simulink model "verification"  (R2015b)
settings: Solver=VariableStepAuto  StartTime=0.0  StopTime=inf  RelTol=1e-3
libraries: neural x20, visionsinks x2, visionstatistics x1
(part 1 of 3)
settings Model: Creator=User  LastModifiedBy=User

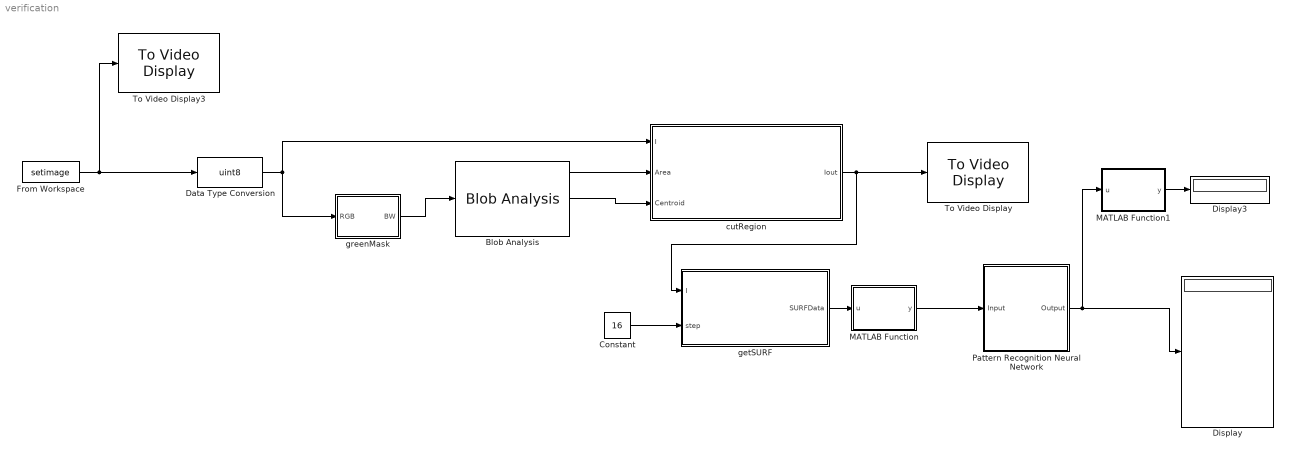
== system verification ==
  Blob Analysis : visionstatistics/Blob Analysis  Tag=vipblks_row_conv  area=on  centroid=on  bBox=on  majorAxis=off  minorAxis=off  angle=off  eccentricity=off  equivDiameterSq=off  extent=off  perimeter=off  maxBlobs=10  warnIfNumBlobsExceeded=on  isCount=off  useMinArea=off  minArea=0  useMaxArea=off  maxArea=intmax('uint32')  excludeBorderBlob=off  outDT=double  isOutVarDim=off  isFill=on  fillValues=-1  conn=8  isLabel=off  outputMode=Binary point scaling  outputWordLength=32  outputFracLength=16  firstCoeffMode=Binary point scaling  firstCoeffWordLength=16  firstCoeffFracLength=14  secondCoeffMode=Binary point scaling  secondCoeffWordLength=32  secondCoeffFracLength=16  accumMode=Binary point scaling  accumWordLength=32  accumFracLength=0  prodOutputMode=Binary point scaling  prodOutputWordLength=32  prodOutputFracLength=16  roundingMode=Floor  overflowMode=off
  Constant : Constant  Value=16
  Data Type Conversion : DataTypeConversion  OutDataTypeStr=uint8
  Display : Display
  Display3 : Display
  From Workspace : FromWorkspace  VariableName=setimage  SampleTime=2  Interpolate=off  OutputAfterFinalValue=Setting to zero
  MATLAB Function : MATLAB Function  TreatAsAtomicUnit=on
  MATLAB Function1 : MATLAB Function  TreatAsAtomicUnit=on
  Pattern Recognition Neural Network : Subsystem
      mask help: Pattern Recognition Neural Network
      mask Display: e = 0.06;c1 = [120 150 230]/255;c2 = ([120 150 230]+0)/383;c3 = ([120 150 230]+128)/383;patch([0 1 1 0],[0 0 1 1],c1);patch([0 1 1 1-e 1-e 0+e],[0 0 1 1-e 0+e 0+e],c2);patch([0 0 1 1-e 0+e 0+e],[0 1 1 1-e 1-e 0+e],c3);plot([0 1 1 0 0],[0 0 1 1 0]);fprintf('NNET');port_label('input',1,' Input');port_label('output',1,'Output ');
  To Video Display : visionsinks/To Video Display  windowSizeMode=Normal  openAtMdlStart=on  fullScreen=off  videoWindowX=1478  videoWindowY=273  saveWindowSize=off  videoWindowWidth=160  videoWindowHeight=160  inputColorFormat=RGB  inputType=Obsolete  imagePorts=One multidimensional signal  OutputDevice=On-screen video monitor  dataOrg=Column-major  isWindowOpen=off
  To Video Display3 : visionsinks/To Video Display  windowSizeMode=Normal  openAtMdlStart=on  fullScreen=off  videoWindowX=536805376  videoWindowY=536805376  saveWindowSize=off  videoWindowWidth=2147483647  videoWindowHeight=2147483647  inputColorFormat=RGB  inputType=Obsolete  imagePorts=One multidimensional signal  OutputDevice=On-screen video monitor  dataOrg=Column-major  isWindowOpen=off
  cutRegion : MATLAB Function  TreatAsAtomicUnit=on
  getSURF : MATLAB Function  TreatAsAtomicUnit=on
  greenMask : MATLAB Function  TreatAsAtomicUnit=on
  wires:
  greenMask/1(BW) -> Blob Analysis/1
  Blob Analysis/2 -> cutRegion/3(Centroid)
  Blob Analysis/1 -> cutRegion/2(Area)
  Constant/1 -> getSURF/2(step)
  cutRegion/1(Iout) -> To Video Display/1, getSURF/1(I)
  Data Type Conversion/1 -> cutRegion/1(I), greenMask/1(RGB)
  getSURF/1(SURFData) -> MATLAB Function/1(u)
  MATLAB Function/1(y) -> Pattern Recognition Neural Network/1(Input)
  From Workspace/1 -> To Video Display3/1, Data Type Conversion/1
  Pattern Recognition Neural Network/1(Output) -> MATLAB Function1/1(u), Display/1
  MATLAB Function1/1(y) -> Display3/1

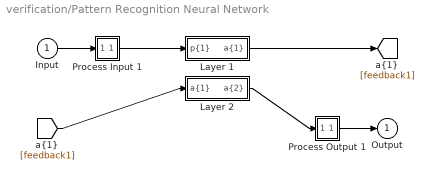
== system verification/Pattern Recognition Neural Network ==
  Input : Inport  PortDimensions=349
      mask Display: e = 0.06;c1 = [120 230 180]/255;c2 = ([120 230 180]+0)/(256+128);c3 = ([120 230 180]+128)/(256+128);patch([0 1 1 0],[0 0 1 1],c1);patch([0 1 1 1-e 1-e 0+e],[0 0 1 1-e 0+e 0+e],c2);patch([0 0 1 1-e 0+e 0+e],[0 1 1 1-e 1-e 0+e],c3);plot([0 1 1 0 0],[0 0 1 1 0]);
  Layer 1 : Subsystem
      mask Display: e = 0.06;c1 = [120 150 230]/255;c2 = ([120 150 230]+0)/383;c3 = ([120 150 230]+128)/383;patch([0 1 1 0],[0 0 1 1],c1);patch([0 1 1 1-e 1-e 0+e],[0 0 1 1-e 0+e 0+e],c2);patch([0 0 1 1-e 0+e 0+e],[0 1 1 1-e 1-e 0+e],c3);plot([0 1 1 0 0],[0 0 1 1 0]);
  Layer 2 : Subsystem
      mask Display: e = 0.06;c1 = [120 150 230]/255;c2 = ([120 150 230]+0)/383;c3 = ([120 150 230]+128)/383;patch([0 1 1 0],[0 0 1 1],c1);patch([0 1 1 1-e 1-e 0+e],[0 0 1 1-e 0+e 0+e],c2);patch([0 0 1 1-e 0+e 0+e],[0 1 1 1-e 1-e 0+e],c3);plot([0 1 1 0 0],[0 0 1 1 0]);
  Process Input 1 : Subsystem
      mask Display: e = 0.06;c1 = [120 150 230]/255;c2 = ([120 150 230]+0)/383;c3 = ([120 150 230]+128)/383;patch([0 1 1 0],[0 0 1 1],c1);patch([0 1 1 1-e 1-e 0+e],[0 0 1 1-e 0+e 0+e],c2);patch([0 0 1 1-e 0+e 0+e],[0 1 1 1-e 1-e 0+e],c3);plot([0 1 1 0 0],[0 0 1 1 0]);
  Process Output 1 : Subsystem
      mask Display: e = 0.06;c1 = [120 150 230]/255;c2 = ([120 150 230]+0)/383;c3 = ([120 150 230]+128)/383;patch([0 1 1 0],[0 0 1 1],c1);patch([0 1 1 1-e 1-e 0+e],[0 0 1 1-e 0+e 0+e],c2);patch([0 0 1 1-e 0+e 0+e],[0 1 1 1-e 1-e 0+e],c3);plot([0 1 1 0 0],[0 0 1 1 0]);
  Output : Outport  InitialOutput=[0;0;0;0;0;0;0]
      mask Display: e = 0.06;c1 = [120 230 180]/255;c2 = ([120 230 180]+0)/(256+128);c3 = ([120 230 180]+128)/(256+128);patch([0 1 1 0],[0 0 1 1],c1);patch([0 1 1 1-e 1-e 0+e],[0 0 1 1-e 0+e 0+e],c2);patch([0 0 1 1-e 0+e 0+e],[0 1 1 1-e 1-e 0+e],c3);plot([0 1 1 0 0],[0 0 1 1 0]);
  wires:
  Input/1 -> Process Input 1/1(x)
  Process Output 1/1(y) -> Output/1
  Process Input 1/1(p) -> Layer 1/1("p{1}")
  Layer 1/1("a{1}") -> [feedback1]
  [feedback1] -> Layer 2/1("a{1} ")
  Layer 2/1("a{2}") -> Process Output 1/1(a)

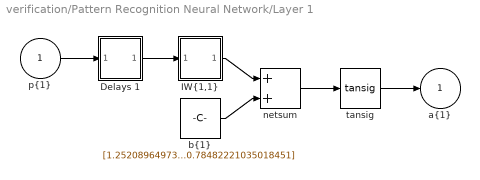
== system verification/Pattern Recognition Neural Network/Layer 1 ==
  "p{1}" : Inport  PortDimensions=349
      mask Display: e = 0.06;c1 = [120 230 180]/255;c2 = ([120 230 180]+0)/(256+128);c3 = ([120 230 180]+128)/(256+128);patch([0 1 1 0],[0 0 1 1],c1);patch([0 1 1 1-e 1-e 0+e],[0 0 1 1-e 0+e 0+e],c2);patch([0 0 1 1-e 0+e 0+e],[0 1 1 1-e 1-e 0+e],c3);plot([0 1 1 0 0],[0 0 1 1 0]);
  Delays 1 : Subsystem
      mask Display: e = 0.06;c1 = [120 150 230]/255;c2 = ([120 150 230]+0)/383;c3 = ([120 150 230]+128)/383;patch([0 1 1 0],[0 0 1 1],c1);patch([0 1 1 1-e 1-e 0+e],[0 0 1 1-e 0+e 0+e],c2);patch([0 0 1 1-e 0+e 0+e],[0 1 1 1-e 1-e 0+e],c3);plot([0 1 1 0 0],[0 0 1 1 0]);disp('0');
  "IW{1,1}" : Subsystem
      mask Display: e = 0.06;c1 = [120 150 230]/255;c2 = ([120 150 230]+0)/383;c3 = ([120 150 230]+128)/383;patch([0 1 1 0],[0 0 1 1],c1);patch([0 1 1 1-e 1-e 0+e],[0 0 1 1-e 0+e 0+e],c2);patch([0 0 1 1-e 0+e 0+e],[0 1 1 1-e 1-e 0+e],c3);plot([0 1 1 0 0],[0 0 1 1 0]);disp('W');
  "b{1}" : Constant  Value=[1.2520896497359288;-0.92281616914926501;-1.5755720804159823;-0.48231286693993536;0.032429505453323522;-0.10257136982966432;0.079130367651085678;0.67536543039361374;0.53417313742188333;0.78482221035018451]
      mask Display: e = 0.06;c1 = [120 150 230]/255;c2 = ([120 150 230]+0)/383;c3 = ([120 150 230]+128)/383;patch([0 1 1 0],[0 0 1 1],c1);patch([0 1 1 1-e 1-e 0+e],[0 0 1 1-e 0+e 0+e],c2);patch([0 0 1 1-e 0+e 0+e],[0 1 1 1-e 1-e 0+e],c3);plot([0 1 1 0 0],[0 0 1 1 0]);disp('b');
  netsum : Sum  Inputs=2  SaturateOnIntegerOverflow=on  InputSameDT=on  OutDataTypeStr=Inherit: Same as first input
      mask Display: e = 0.06;c1 = [120 150 230]/255;c2 = ([120 150 230]+0)/383;c3 = ([120 150 230]+128)/383;patch([0 1 1 0],[0 0 1 1],c1);patch([0 1 1 1-e 1-e 0+e],[0 0 1 1-e 0+e 0+e],c2);patch([0 0 1 1-e 0+e 0+e],[0 1 1 1-e 1-e 0+e],c3);plot([0 1 1 0 0],[0 0 1 1 0]);disp('+');
  tansig : neural/Transfer Functions/tansig
  "a{1}" : Outport  InitialOutput=[0;0;0;0;0;0;0;0;0;0]
      mask Display: e = 0.06;c1 = [120 230 180]/255;c2 = ([120 230 180]+0)/(256+128);c3 = ([120 230 180]+128)/(256+128);patch([0 1 1 0],[0 0 1 1],c1);patch([0 1 1 1-e 1-e 0+e],[0 0 1 1-e 0+e 0+e],c2);patch([0 0 1 1-e 0+e 0+e],[0 1 1 1-e 1-e 0+e],c3);plot([0 1 1 0 0],[0 0 1 1 0]);
  wires:
  "p{1}"/1 -> Delays 1/1("p{1}")
  Delays 1/1("pd{1,1}") -> "IW{1,1}"/1("pd{1,1}")
  "IW{1,1}"/1("iz{1,1}") -> netsum/1
  "b{1}"/1 -> netsum/2
  netsum/1 -> tansig/1
  tansig/1 -> "a{1}"/1

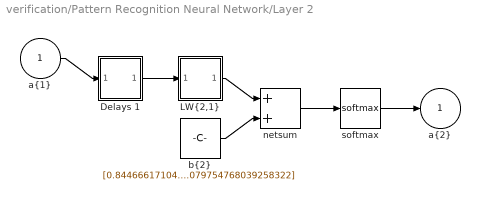
== system verification/Pattern Recognition Neural Network/Layer 2 ==
  "a{1} " : Inport  PortDimensions=10
      mask Display: e = 0.06;c1 = [120 230 180]/255;c2 = ([120 230 180]+0)/(256+128);c3 = ([120 230 180]+128)/(256+128);patch([0 1 1 0],[0 0 1 1],c1);patch([0 1 1 1-e 1-e 0+e],[0 0 1 1-e 0+e 0+e],c2);patch([0 0 1 1-e 0+e 0+e],[0 1 1 1-e 1-e 0+e],c3);plot([0 1 1 0 0],[0 0 1 1 0]);
  Delays 1 : Subsystem
      mask Display: e = 0.06;c1 = [120 150 230]/255;c2 = ([120 150 230]+0)/383;c3 = ([120 150 230]+128)/383;patch([0 1 1 0],[0 0 1 1],c1);patch([0 1 1 1-e 1-e 0+e],[0 0 1 1-e 0+e 0+e],c2);patch([0 0 1 1-e 0+e 0+e],[0 1 1 1-e 1-e 0+e],c3);plot([0 1 1 0 0],[0 0 1 1 0]);disp('0');
  "LW{2,1}" : Subsystem
      mask Display: e = 0.06;c1 = [120 150 230]/255;c2 = ([120 150 230]+0)/383;c3 = ([120 150 230]+128)/383;patch([0 1 1 0],[0 0 1 1],c1);patch([0 1 1 1-e 1-e 0+e],[0 0 1 1-e 0+e 0+e],c2);patch([0 0 1 1-e 0+e 0+e],[0 1 1 1-e 1-e 0+e],c3);plot([0 1 1 0 0],[0 0 1 1 0]);disp('W');
  "b{2}" : Constant  Value=[0.8446661710451735;-0.96183712929880982;0.74210025390233625;0.16753901818095251;-0.54254157655283242;-0.63817454211815539;-0.079754768039258322]
      mask Display: e = 0.06;c1 = [120 150 230]/255;c2 = ([120 150 230]+0)/383;c3 = ([120 150 230]+128)/383;patch([0 1 1 0],[0 0 1 1],c1);patch([0 1 1 1-e 1-e 0+e],[0 0 1 1-e 0+e 0+e],c2);patch([0 0 1 1-e 0+e 0+e],[0 1 1 1-e 1-e 0+e],c3);plot([0 1 1 0 0],[0 0 1 1 0]);disp('b');
  netsum : Sum  Inputs=2  SaturateOnIntegerOverflow=on  InputSameDT=on  OutDataTypeStr=Inherit: Same as first input
      mask Display: e = 0.06;c1 = [120 150 230]/255;c2 = ([120 150 230]+0)/383;c3 = ([120 150 230]+128)/383;patch([0 1 1 0],[0 0 1 1],c1);patch([0 1 1 1-e 1-e 0+e],[0 0 1 1-e 0+e 0+e],c2);patch([0 0 1 1-e 0+e 0+e],[0 1 1 1-e 1-e 0+e],c3);plot([0 1 1 0 0],[0 0 1 1 0]);disp('+');
  softmax : neural/Transfer Functions/softmax
  "a{2}" : Outport  InitialOutput=[0;0;0;0;0;0;0]
      mask Display: e = 0.06;c1 = [120 230 180]/255;c2 = ([120 230 180]+0)/(256+128);c3 = ([120 230 180]+128)/(256+128);patch([0 1 1 0],[0 0 1 1],c1);patch([0 1 1 1-e 1-e 0+e],[0 0 1 1-e 0+e 0+e],c2);patch([0 0 1 1-e 0+e 0+e],[0 1 1 1-e 1-e 0+e],c3);plot([0 1 1 0 0],[0 0 1 1 0]);
  wires:
  "a{1} "/1 -> Delays 1/1("p{2}")
  Delays 1/1("pd{2,1}") -> "LW{2,1}"/1("ad{2,1}")
  "LW{2,1}"/1("lz{2,1}") -> netsum/1
  "b{2}"/1 -> netsum/2
  netsum/1 -> softmax/1
  softmax/1 -> "a{2}"/1

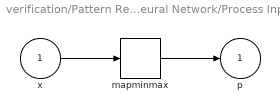
== system verification/Pattern Recognition Neural Network/Process Input 1 ==
  x : Inport  PortDimensions=349
      mask Display: e = 0.06;c1 = [120 230 180]/255;c2 = ([120 230 180]+0)/(256+128);c3 = ([120 230 180]+128)/(256+128);patch([0 1 1 0],[0 0 1 1],c1);patch([0 1 1 1-e 1-e 0+e],[0 0 1 1-e 0+e 0+e],c2);patch([0 0 1 1-e 0+e 0+e],[0 1 1 1-e 1-e 0+e],c3);plot([0 1 1 0 0],[0 0 1 1 0]);
  mapminmax : neural/Processing Functions/mapminmax  xmin=[-11129.965961101443;1134.6567206044926;-2376.3659908917143;-4334.0372445314288;7757.4027746883612;-6984.4334074929839;-2777.9527058342687;3155.9690581192376;-1330.691241389575;4257.0589253908138;-623.20684359631468;-2001.566675005465;-4932.7134689911391;304.46851647603125;-967.32875854233816;640.73136885648694;386.66074504769114;1002.1623313175693;-3184.007659381773;-381.37803132283284;-3295.858092291508;-1489.0871261009588;-226.49555101296443;-2405.8867516242576;-2776.7794520500211;-1541.0170324268913;101.43967602768807;-100.76443127754578;-593.03637636096903;1357.9634170740264;1407.3950263055601;-483.66947575357494;-1889.9176508706948;-1629.3955251451089;-726.50327548468738;-1853.6072505650598;-1498.8553267377129;-1530.3633390778268;268.18750457084093;-2240.9999713540606;-1598.6795958119494;-1582.907954987654;380.23677697560817;-687.57622036680209;-2158.6653002343019;-1530.8506902527345;-2225.7407166340577;-1737.1719827748605;386.28554587051292;-2047.1309669819805;-1417.8656347977224;-612.48056407820786;676.45691636688923;446.38920725912357;74.470862862096908;39.174713487048386;-1007.1653257389228;-1067.5381147129376;-1589.7717010748245;369.32541111978048;-15.568258331743834;-2618.166478036178;66.851725230876625;-2632.6489110914567;-152.27189245653938;-961.70356716324886;-68.16047275108798;-1389.6973712632755;-1544.6280829615475;-1078.1701102250183;-1083.2475056257147;-70.327106602471815;-1389.6912572643412;-501.87203323128261;-1211.1299730501946;-873.8563577745025;135.23078707803614;510.40761207152661;67.976583540881691;-382.71067889430486;-2440.8434161611667;-960.30021713058647;601.55410753465776;-920.69305223222057;-945.98625046016025;-1158.0540952187496;260.30244378313034;-1087.9748915817286;-582.19629937786613;-494.80610196790803;-1423.8822861380806;-1415.6427970118482;-589.82126941908848;66.389992254750979;-1287.5678718628087;-40.246203034889106;-1450.5155667211093;-697.93893844304534;-121.38825064237872;-1029.850343236707;-258.78167810452703;-1184.1571756240155;-175.02600935248478;-1173.3831276484862;-845.55385054668193;-1118.0261569261522;-112.80399351655041;285.29099479332041;-406.88257108720899;-824.4577050291407;-913.16225540445407;-431.74577653476297;-535.29039798765666;-559.55309131633362;-859.66088958315208;-1382.5184253003295;-634.44889621500624;-869.9885065509344;-1736.0447306117053;-989.43057866603237;-377.04364635953357;-655.34244197384805;-1161.4001166516846;-354.69697407530305;-410.240777822631;-763.08944947808925;-882.01049096338215;-17.297235561955929;-853.68060261106541;-388.55640302193973;260.40063239144388;-614.33797117366726;-1166.0372444888003;-829.31885826600205;-1106.1198195175425;-117.14159077934548;172.43508067231105;-269.31758186795628;-1189.4586228827602;-585.82582165939368;-296.54465016092115;-1217.9356712043461;-425.125346288532;-956.89102108175575;130.81562066503227;-650.61070961528071;-35.453495601084455;-374.16957679196389;-756.19410654695184;-436.24479084948632;-166.7746883075414;-402.54135427924291;-1012.3923778324571;-448.67046874191061;-288.18820186606865;-99.014151169624313;-160.80695606286076;-521.75050070627856;-565.41663842242019;-576.59406290264189;-778.2488779178459;-1366.4710747970648;-368.11986679262969;-470.81863934027433;-314.58819838502666;-766.97148873280241;-468.21981709565682;-120.09837788639067;-936.80795693703726;-574.10147881344369;-556.44364225382867;-101.95169318831634;-292.5992032047817;-1077.7752146961855;461.34208371091569;492.30461418312234;-62.101593456599197;-277.72177129517496;-715.16524137409272;-820.91429927317392;-403.25066908313806;-354.19848681396775;-328.28100657612879;-606.65121012463112;-723.6632390586019;-126.01168221322104;496.64864785796067;-527.94553740683682;-76.910242259943942;-213.85663435464679;-291.10212552221253;-693.61749700215705;-718.36036545535615;-470.16860826413154;-507.09195521529062;-24.160913119847585;-356.3012042668787;-110.1797003545517;-257.23099780974258;-493.00999691856509;-413.53664259676259;359.44871453975867 ...(+2909 chars)]  xmax=[397.78167723661954;8436.3912606232279;5867.9385092102521;6311.2023660377272;15916.678863228881;-1313.2793983486183;2315.3067312547978;8728.7337071799957;2875.8975677575868;9991.0214449512478;4512.8412251466652;2355.8137600612786;-1408.6126422904806;3496.7337572167885;2224.3238892180129;3513.4113452470406;3953.658351406958;4805.6948482318785;449.31688747905389;2253.5991045715514;-165.95112097420241;1389.1057537491156;2332.4274940169826;295.64512590558331;237.33551059239605;962.14719666108783;2977.9432266360059;2737.8278146943221;1561.5716819504321;3405.1461090272451;3027.3017757628427;1624.166135001152;517.02495743458167;579.89400277239884;2067.7743115093072;-174.73747439593853;45.940031745344541;1082.5545645494383;2057.2578601041027;287.97406840136239;-7.4682838646715695;230.95918445091701;2176.0860746235198;1863.1704702582781;-360.65582537058845;609.4552644082421;-595.85660678728698;22.967508257476101;2214.175477912207;-327.44982267284752;381.54237479419544;1144.6522986243888;2255.9618454314391;1961.8729426624452;1669.4073114653456;1493.9835504704438;945.06349258273076;853.26185953532968;-350.08394451167248;1938.9787479497484;1296.0526686651579;-1297.5161435056723;1413.1199356927327;-1397.4668194636049;1203.7361519000365;414.33194305704717;1158.4931674465781;4.3213942425819454;-257.16139149441898;121.14492732889181;43.602565149757524;1289.7268332030173;-121.5089895600681;845.25454281981149;3.6335637431844248;297.79121185655015;1288.9893899466165;1792.4780980246187;1293.7173988137965;871.45997126634677;-1206.0990251770727;180.9681255538261;1803.8357580198731;184.44920406903697;66.276190621532422;-175.57942918644488;1253.4470671572942;106.37391764225229;402.75085040828276;544.3990508048804;9.1184833703907771;-301.04350600765918;507.75693571125527;1206.9329633433083;-400.69933146410864;792.42940136847039;-286.09713029253322;359.00538717727022;1227.0886861476365;-94.317579624405198;822.61715472861079;-311.65308075708157;658.98228750215924;-281.88468181579259;178.64673981753467;-48.810510618512154;1001.1476763257616;1069.9772101902463;434.35115999108518;-20.164617294489261;121.23890660250443;439.21325674879677;363.19411212891913;270.06403402609504;-17.709692640582077;-400.50658988500572;307.91071085810017;59.888279361453684;-849.17600388234644;-222.43316776665415;406.34050546514459;77.72389833803355;-369.62088836929337;340.01951858772827;679.85557020579711;-12.120606205952711;-161.29266901927809;846.62310938045084;51.464443248133861;297.22194419031939;1022.7351843319689;332.85998436330789;-397.23107112965079;61.092835054348129;-453.58651099189808;553.45123096273653;954.17267774755373;406.65698690545281;-469.10265295533958;184.14813323426839;334.61261109401664;-581.51335210944558;249.14593449043156;-368.36951144813139;763.39570625902991;-3.1675987086032933;643.00853593280794;361.67556567385162;-30.240265588781384;291.51782292413162;604.69781743434237;441.73255135020906;-436.44071122764774;429.33782806111748;417.25229830393653;508.41888985176439;610.58421231244961;134.90182379508144;45.021111482170028;187.51685860073817;-121.83047292404831;-708.18044063738341;127.13667924827588;352.07319598987118;253.30489311026201;-96.998432264900003;130.78400181618275;585.61778495745705;-379.57002124574586;37.989116649839133;206.28837492859287;523.59054371327068;240.10293720178657;-350.82844372115943;1016.4353244600668;1000.0645970904562;504.24418552918883;370.94951893509699;-178.93253116683363;-196.09657167509781;244.51537310454421;146.10241204340969;166.50597996521708;-16.252871801035575;-101.83744206441233;435.82225856850414;1075.7743063014293;70.559257694180928;487.94045762198436;330.17599179875538;216.73919879644518;-87.763675964587392;-72.050092264330445;55.300787432147573;10.935217805300226;530.33352701332706;112.52503956863384;425.34336304997169;258.21418181897138;6.0875771904963401;145.36322628448636;919.07312170914986;-237.06580224356924;-208.87876743628652;521.37416361842497;508.08819503435359;-122.7431759592109;305.86485607225546 ...(+2708 chars)]  ymin=-1  ymax=1
  p : Outport  PortDimensions=349
      mask Display: e = 0.06;c1 = [120 230 180]/255;c2 = ([120 230 180]+0)/(256+128);c3 = ([120 230 180]+128)/(256+128);patch([0 1 1 0],[0 0 1 1],c1);patch([0 1 1 1-e 1-e 0+e],[0 0 1 1-e 0+e 0+e],c2);patch([0 0 1 1-e 0+e 0+e],[0 1 1 1-e 1-e 0+e],c3);plot([0 1 1 0 0],[0 0 1 1 0]);
  wires:
  x/1 -> mapminmax/1
  mapminmax/1 -> p/1

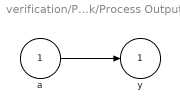
== system verification/Pattern Recognition Neural Network/Process Output 1 ==
  a : Inport  PortDimensions=7
      mask Display: e = 0.06;c1 = [120 230 180]/255;c2 = ([120 230 180]+0)/(256+128);c3 = ([120 230 180]+128)/(256+128);patch([0 1 1 0],[0 0 1 1],c1);patch([0 1 1 1-e 1-e 0+e],[0 0 1 1-e 0+e 0+e],c2);patch([0 0 1 1-e 0+e 0+e],[0 1 1 1-e 1-e 0+e],c3);plot([0 1 1 0 0],[0 0 1 1 0]);
  y : Outport  PortDimensions=7
      mask Display: e = 0.06;c1 = [120 230 180]/255;c2 = ([120 230 180]+0)/(256+128);c3 = ([120 230 180]+128)/(256+128);patch([0 1 1 0],[0 0 1 1],c1);patch([0 1 1 1-e 1-e 0+e],[0 0 1 1-e 0+e 0+e],c2);patch([0 0 1 1-e 0+e 0+e],[0 1 1 1-e 1-e 0+e],c3);plot([0 1 1 0 0],[0 0 1 1 0]);
  wires:
  a/1 -> y/1

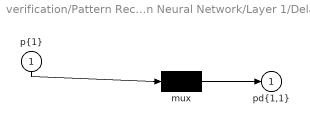
== system verification/Pattern Recognition Neural Network/Layer 1/Delays 1 ==
  "p{1}" : Inport  PortDimensions=349
      mask Display: e = 0.06;c1 = [120 230 180]/255;c2 = ([120 230 180]+0)/(256+128);c3 = ([120 230 180]+128)/(256+128);patch([0 1 1 0],[0 0 1 1],c1);patch([0 1 1 1-e 1-e 0+e],[0 0 1 1-e 0+e 0+e],c2);patch([0 0 1 1-e 0+e 0+e],[0 1 1 1-e 1-e 0+e],c3);plot([0 1 1 0 0],[0 0 1 1 0]);
  mux : Mux  Inputs=1
      mask Display: e = 0.06;c1 = [120 150 230]/255;c2 = ([120 150 230]+0)/383;c3 = ([120 150 230]+128)/383;patch([0 1 1 0],[0 0 1 1],c1);patch([0 1 1 1-e 1-e 0+e],[0 0 1 1-e 0+e 0+e],c2);patch([0 0 1 1-e 0+e 0+e],[0 1 1 1-e 1-e 0+e],c3);plot([0 1 1 0 0],[0 0 1 1 0]);disp('Mux')
  "pd{1,1}" : Outport
      mask Display: e = 0.06;c1 = [120 230 180]/255;c2 = ([120 230 180]+0)/(256+128);c3 = ([120 230 180]+128)/(256+128);patch([0 1 1 0],[0 0 1 1],c1);patch([0 1 1 1-e 1-e 0+e],[0 0 1 1-e 0+e 0+e],c2);patch([0 0 1 1-e 0+e 0+e],[0 1 1 1-e 1-e 0+e],c3);plot([0 1 1 0 0],[0 0 1 1 0]);
  wires:
  "p{1}"/1 -> mux/1
  mux/1 -> "pd{1,1}"/1
